simulink model "vehicle_animation_sim"  (Simulink 8.8)
settings: Solver=ode45  StartTime=0.0  StopTime=154  RelTol=1e-3  EnableMultiTasking=on
values from neighbouring files (symbols this model uses):
  vehicle_length = 2    [setup.m]
  X_ic = 0    [setup.m]
  Y_ic = 0    [setup.m]
  yaw_ic = 1*(-pi/2)    (= -1.57079632679)    [setup.m]
undefined symbols (not defined in the file): animation_update_interval, datetime, enable_CG_trace, enable_rearAxle_trace, plotAxisLimitMode, plotAxisLimits, save_anim_frames, vehicle_width
libraries: simulink x2
settings Model: Creator=comperem  LastModifiedBy=Administrator
settings DataIOCC: SignalLoggingSaveFormat=Dataset
settings OptimizationCC: BlockReduction=off  BooleanDataType=off
settings DebuggingCC: SaveWithParameterizedLinksMsg=none  SignalResolutionControl=TryResolveAllWithWarning  FcnCallInpInsideContextMsg=error  AllowSymbolicDim=off  StateNameClashWarn=none
settings HardwareCC: TargetUnknown=on
settings RTWCC: TargetLang=C++
settings GRTTargetCC: CombineOutputUpdateFcns=on  MultiInstanceERTCode=on  CodeInterfacePackaging=C++ class  GRTInterface=off
settings CPPComponent: GenerateDestructor=on  GenerateExternalIOAccessMethods=None  ParameterMemberVisibility=private  InternalMemberVisibility=private  GenerateParameterAccessMethods=None  GenerateInternalMemberAccessMethods=None  UseOperatorNewForModelRefRegistration=off
settings ConfigComp: CovSFcnEnable=off

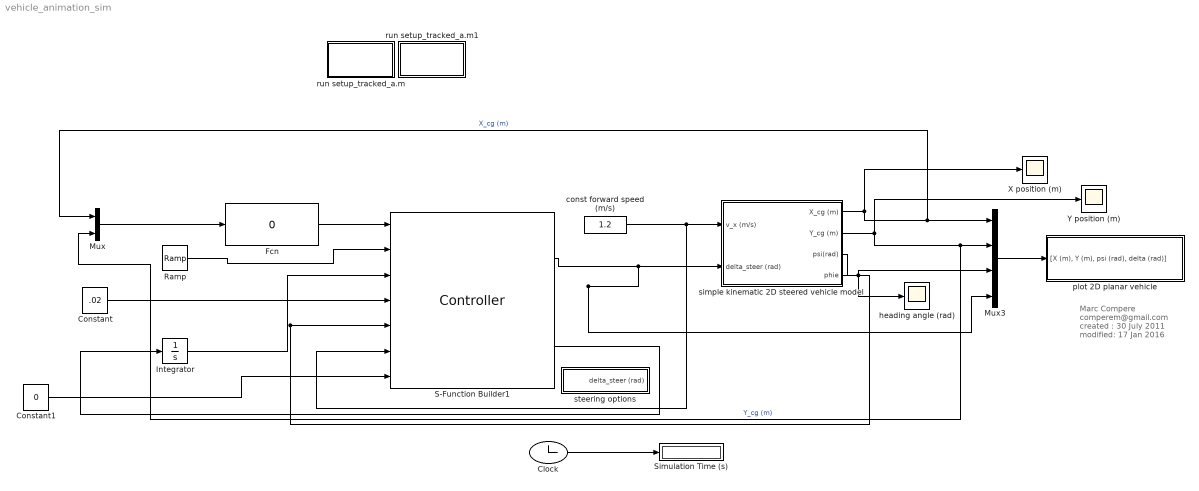
== system vehicle_animation_sim ==
  note: Marc Compere
      | comperem@gmail.com
      | created : 30 July 2011
      | modified: 17 Jan 2016
  Clock : Clock
      settings: Decimation=50
  Constant : Constant  Value=.02
  Constant1 : Constant  Value=0
  Fcn : Fcn  Expr=0
  Integrator : Integrator
  Mux : Mux  Inputs=2
  Mux3 : Mux
  Ramp : simulink/Sources/Ramp  slope=.02  start=0  X0=0.1
  S-Function Builder1 : S-Function  InitFcn=try, set_param(gcb,'FunctionName','Controller'), end  FunctionName=Controller  Parameters=1,3,3,vehicle_length  SFunctionModules=Controller_wrapper  WizardData=DataTag0  SFunctionDeploymentMode=off  EnableBusSupport=off  mask(S-Function Builder){}
      mask help: Simulink:masks:SFunctionBuilder_MD
      mask init:
      | val = [[.9  0.75 0.75 1 1 .9 .9 1]',[1 1 0.75 0.75 .9 .9 1 .9]'];try , sys = get_param(gcb,'SfunBuilderFcnName');if isempty(sys), sys = get_param(gcb,'FunctionName'); end,catch, sys = get_param(gcb,'FunctionName'); end
      settings: CopyFcn=set_param(gcbh,'LinkStatus','none')  PreSaveFcn=try, set_param(gcb,'FunctionName','Controller'), end  OpenFcn=sfunctionwizard(gcbh)
      mask Display: plot(val(:,1),val(:,2)),disp(sys), port_label('input',1,'d'), port_label('input',2,'thetaE'), port_label('input',3,'s'), port_label('input',4,'cS'), port_label('input',5,'phie'), port_label('input',6,'u1'), port_label('input',7,'cDE'), port_label('output',1,'v2'), port_label('output',2,'V1')
  Simulation Time (s) : Display
      settings: Format=short_e  Decimation=5
  X position (m) : Scope
  Y position (m) : Scope
  const forward speed (m/s) : Constant  Value=1.2
  heading angle (rad) : Scope
  plot 2D planar vehicle : Subsystem  mask(6DoF Animation){axisMode=plotAxisLimitMode, ax=plotAxisLimits, Ts=animation_update_interval, enable_CG_trace=enable_CG_trace, enable_rearAxle_trace=enable_rearAxle_trace, save_anim_frames=save_anim_frames, anim_frame_name_str=char(datetime('now','Format','yyyy-MM-dd_HH_mm_ss')), L=vehicle_length, W=vehicle_width}
      mask prompts: axisMode "Axis Mode (0->auto, 1->fixed, BOTH use Axes Limits below)"; ax "Axes limits [xmin xmax ymin ymax] (m):"; Ts "Time interval between updates (s):"; enable_CG_trace "Enable vehicle CG trace? (0/1)"; enable_rearAxle_trace "Enable rear axle trace? (0/1)"; save_anim_frames "Save animaton frames? (0/1)"; anim_frame_name_str "Animation sequence name (if save frames==1)"; L "Vehicle length (m)"; W "Vehicle width (m)"
      mask help:
      | Create a 2D animated view of a steering vehicle model with tires.
      |
      | Marc Compere
      | CompereM@saic.com
      | created : 22 August 2002
      | modified: 28 Dec 2015
      mask init:
      | Config.axisMode=axisMode;
      | Config.ax=ax;
      | Config.Ts=Ts;
      | Config.enable_CG_trace=enable_CG_trace;
      | Config.enable_rearAxle_trace=enable_rearAxle_trace;
      | Config.save_anim_frames=save_anim_frames;
      | Config.anim_frame_name_str=anim_frame_name_str;
      | Config.L=L;
      | Config.W=W;
      mask Help:
      | <p>This block generates a 3 dimensional display of a simulation trajectory, with the craft orientation displayed during flight</p>
      | 
      | <p>There are two inputs to this block, Position and Euler.  These inputs contain more than one signal as described below.</p>
      | 
      | <p><H4>Block Vector Input - Position</H4>
      | <ul>
      | <li>X Position</li>
      | <li>Y Position</li>
      | <li>Z Position</li>
      | </ul>
      | </p>
      | 
      | <p><H4>Block Vector Input - Euler</H4>
      |     <ul>
      |     <li>Roll Attitude</li>
      |     <li>Pitch Attitude</li>
      |     <li>Yaw Attitude</li>
      |    </ul>
      |    </p>
  run setup_tracked_a.m : Subsystem
      settings: OpenFcn=setup
      mask Display: fprintf('run setup.m')
  run setup_tracked_a.m1 : Subsystem
      settings: OpenFcn=edit setup
      mask Display: fprintf('edit setup.m')
  simple kinematic 2D steered vehicle model : Subsystem
  steering options : Subsystem
  wires:
  simple kinematic 2D steered vehicle model/1(X_cg (m)) -> Mux/1, Mux3/1, X position (m)/1  "X_cg (m)"
  simple kinematic 2D steered vehicle model/2(Y_cg (m)) -> Mux/2, Mux3/2, Y position (m)/1  "Y_cg (m)"
  const forward speed (m/s)/1 -> S-Function Builder1/6, simple kinematic 2D steered vehicle model/1(v_x (m/s))
  Mux3/1 -> plot 2D planar vehicle/1("[X (m), Y (m), psi (rad), delta (rad)]")
  Clock/1 -> Simulation Time (s)/1
  simple kinematic 2D steered vehicle model/3(psi(rad)) -> heading angle (rad)/1, Mux3/3
  Fcn/1 -> S-Function Builder1/1
  Mux/1 -> Fcn/1
  S-Function Builder1/1 -> Mux3/4, simple kinematic 2D steered vehicle model/2(delta_steer (rad))
  Constant/1 -> S-Function Builder1/4
  Integrator/1 -> S-Function Builder1/3
  S-Function Builder1/2 -> Integrator/1
  Constant1/1 -> S-Function Builder1/7
  simple kinematic 2D steered vehicle model/4(phie) -> S-Function Builder1/5
  Ramp/1 -> S-Function Builder1/2

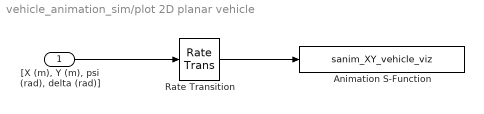
== system vehicle_animation_sim/plot 2D planar vehicle ==
  "[X (m), Y (m), psi (rad), delta (rad)]" : Inport
  Animation S-Function : S-Function  FunctionName=sanim_XY_vehicle_viz  Parameters=Config  SFunctionDeploymentMode=off  EnableBusSupport=off
  Rate Transition : RateTransition  Integrity=off
  wires:
  "[X (m), Y (m), psi (rad), delta (rad)]"/1 -> Rate Transition/1
  Rate Transition/1 -> Animation S-Function/1

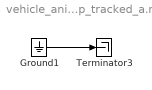
== system vehicle_animation_sim/run setup_tracked_a.m ==
  Ground1 : Ground
  Terminator3 : Terminator
  wires:
  Ground1/1 -> Terminator3/1

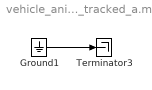
== system vehicle_animation_sim/run setup_tracked_a.m1 ==
  Ground1 : Ground
  Terminator3 : Terminator
  wires:
  Ground1/1 -> Terminator3/1

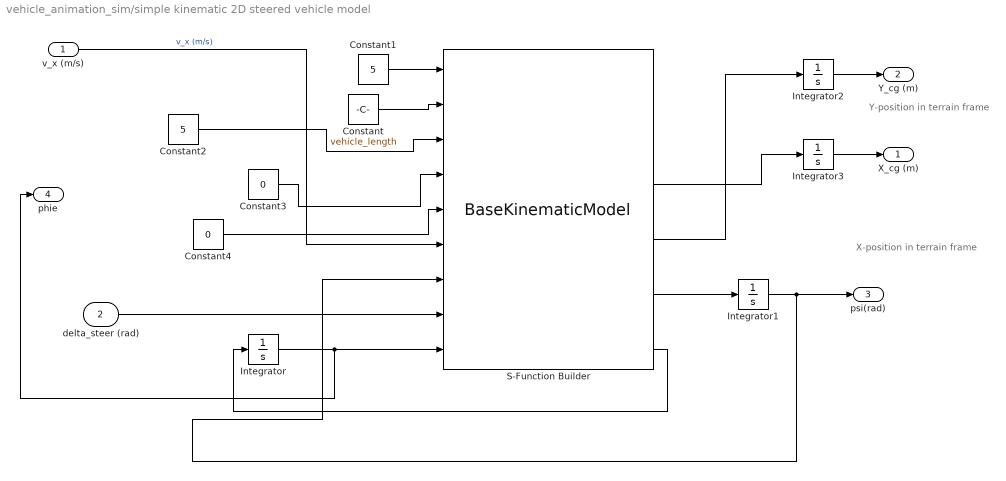
== system vehicle_animation_sim/simple kinematic 2D steered vehicle model ==
  note: X-position in
      | terrain frame
  note: Y-position in
      | terrain frame
  v_x (m/s) : Inport
  delta_steer (rad) : Inport  Port=2
  Constant : Constant  Value=vehicle_length
  Constant1 : Constant  Value=5
  Constant2 : Constant  Value=5
  Constant3 : Constant  Value=0
  Constant4 : Constant  Value=0
  Integrator : Integrator
  Integrator1 : Integrator  InitialCondition=yaw_ic
  Integrator2 : Integrator  InitialCondition=Y_ic
  Integrator3 : Integrator  InitialCondition=X_ic
  S-Function Builder : S-Function  InitFcn=try, set_param(gcb,'FunctionName','BaseKinematicModel'), end  FunctionName=BaseKinematicModel  SFunctionModules=BaseKinematicModel_wrapper  WizardData=DataTag1  SFunctionDeploymentMode=off  EnableBusSupport=off  mask(S-Function Builder){}
      mask help: Simulink:masks:SFunctionBuilder_MD
      mask init: same as vehicle_animation_sim/S-Function Builder1
      settings: CopyFcn=set_param(gcbh,'LinkStatus','none')  PreSaveFcn=try, set_param(gcb,'FunctionName','BaseKinematicModel'), end  OpenFcn=sfunctionwizard(gcbh)
      mask Display: plot(val(:,1),val(:,2)),disp(sys), port_label('input',1,'radius'), port_label('input',2,'length'), port_label('input',3,'distanceLR'), port_label('input',4,'angularVR'), port_label('input',5,'angularVL'), port_label('input',6,'u1'), port_label('input',7,'theta'), port_label('input',8,'u2'), port_label('input',9,'phie'), port_label('output',1,'longVeloc'), port_label('output',2,'rotationalVelocity'), port_label('output',3,'dX'), port_label('output',4,'dY'), port_label('output',5,'dTheta'), port_label('output',6,'dPhie')
  X_cg (m) : Outport
  Y_cg (m) : Outport  Port=2
  psi(rad) : Outport  Port=3
  phie : Outport  Port=4
  wires:
  Integrator3/1 -> X_cg (m)/1
  Integrator2/1 -> Y_cg (m)/1
  S-Function Builder/5 -> Integrator1/1
  Constant1/1 -> S-Function Builder/1
  Constant/1 -> S-Function Builder/2
  Constant2/1 -> S-Function Builder/3
  Constant3/1 -> S-Function Builder/4
  Constant4/1 -> S-Function Builder/5
  delta_steer (rad)/1 -> S-Function Builder/8
  v_x (m/s)/1 -> S-Function Builder/6  "v_x (m/s)"
  Integrator1/1 -> S-Function Builder/7, psi(rad)/1
  S-Function Builder/4 -> Integrator2/1
  S-Function Builder/3 -> Integrator3/1
  Integrator/1 -> phie/1, S-Function Builder/9
  S-Function Builder/6 -> Integrator/1

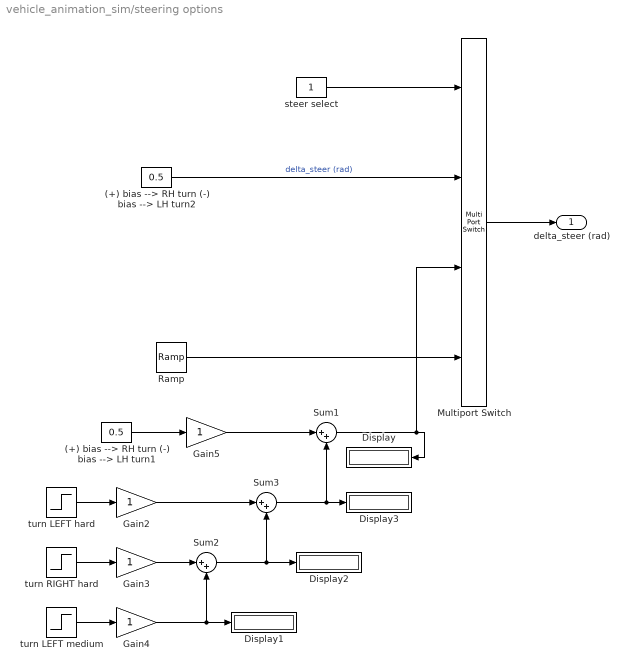
== system vehicle_animation_sim/steering options ==
  (+) bias --> RH turn (-) bias --> LH turn1 : Constant  Value=0.5
  (+) bias --> RH turn (-) bias --> LH turn2 : Constant  Value=0.5
  Display{,1..3} (4 alike) : Display
  Gain{2..5} (4 alike) : Gain
  Multiport Switch : MultiPortSwitch
  Ramp : simulink/Sources/Ramp  slope=.05  start=0  X0=0
  Sum1 : Sum  Inputs=|++
  Sum2 : Sum  Inputs=|++
  Sum3 : Sum  Inputs=|++
  steer select : Constant
  turn LEFT hard : Step  After=-1  SampleTime=0
  turn LEFT medium : Step  After=-0.5  SampleTime=0
  turn RIGHT hard : Step  Time=2  After=+1  SampleTime=0
  delta_steer (rad) : Outport
  wires:
  steer select/1 -> Multiport Switch/1
  Multiport Switch/1 -> delta_steer (rad)/1
  Sum1/1 -> Multiport Switch/3, Display/1
  (+) bias --> RH turn (-) bias --> LH turn1/1 -> Gain5/1
  turn RIGHT hard/1 -> Gain3/1
  turn LEFT medium/1 -> Gain4/1
  turn LEFT hard/1 -> Gain2/1
  Sum2/1 -> Display2/1, Sum3/2
  Sum3/1 -> Display3/1, Sum1/2
  Gain2/1 -> Sum3/1
  Gain3/1 -> Sum2/1
  Gain4/1 -> Display1/1, Sum2/2
  Gain5/1 -> Sum1/1
  (+) bias --> RH turn (-) bias --> LH turn2/1 -> Multiport Switch/2  "delta_steer (rad)"
  Ramp/1 -> Multiport Switch/4
